simulink model "PKE_one_group"  (R2014b)
settings: Solver=ode45  StartTime=0.0  StopTime=10.0  MaxStep=0.01  RelTol=1e-3
settings Model: Creator=VIKRAM SINGH  LastModifiedBy=VIKRAM SINGH
settings SolverCC: InitialStep=0.0001

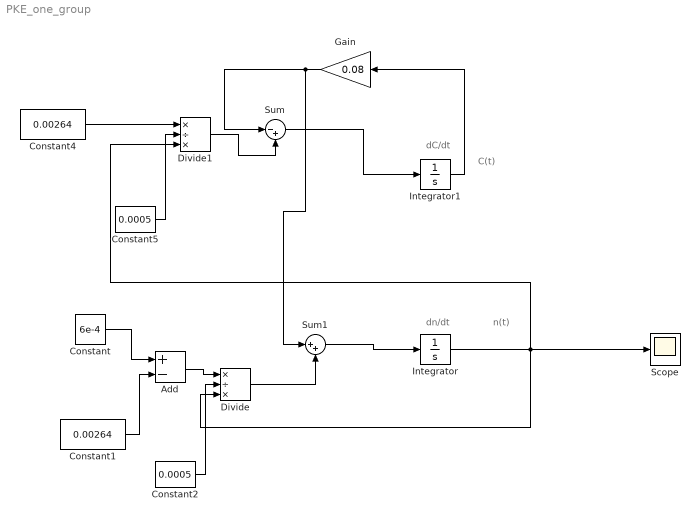
== system PKE_one_group ==
  note: C(t)
  note: dC/dt
  note: dn/dt
  note: n(t)
  Add : Sum  Inputs=+-
  Constant : Constant  Value=6e-4
  Constant1 : Constant  Value=0.00264
  Constant2 : Constant  Value=0.0005
  Constant4 : Constant  Value=0.00264
  Constant5 : Constant  Value=0.0005
  Divide : Product  Inputs=*/*
  Divide1 : Product  Inputs=*/*
  Gain : Gain  Gain=0.08
  Integrator : Integrator  InitialCondition=1.0
  Integrator1 : Integrator  InitialCondition=66.0
  Scope : Scope
  Sum : Sum  Inputs=|-+
  Sum1 : Sum  Inputs=|++
  wires:
  Integrator/1 -> Scope/1, Divide1/3, Divide/3
  Integrator1/1 -> Gain/1
  Constant/1 -> Add/1
  Constant1/1 -> Add/2
  Add/1 -> Divide/1
  Constant2/1 -> Divide/2
  Constant5/1 -> Divide1/2
  Constant4/1 -> Divide1/1
  Gain/1 -> Sum1/1, Sum/1
  Divide1/1 -> Sum/2
  Divide/1 -> Sum1/2
  Sum/1 -> Integrator1/1
  Sum1/1 -> Integrator/1
